simulink model "simu"  (R2025b)
settings: Solver=FixedStepAuto  StartTime=0.0  StopTime=7  FixedStep=0.01  RelTol=1e-3
model workspace (MAT data in the model file):
  T_data = [16.81; 22.34; 22.23; 21.49; 20; 20.21; 18.09; 15.74; 13.4; 10.85; 10.21; 8.94; 8.83; 8.62; 8.62; 8.62; 8.51; 8.72; 8.51; 8.51; 7.77; 7.02; 5.64; 3.83; 2.23; 0.96; 0]
  aero_data.Alpha = [0; 2; 4]
  aero_data.CD = [0.20580088598; 0.20580088598; 0.20580088598]
  aero_data.CL = [0; 0.0625795358549; 0.124860076206]
  aero_data.CP = [0.999; 0.999; 0.999]
  t_data = [0.01; 0.03; 0.11; 0.26; 0.37; 0.47; 0.67; 0.99; 1.31; 1.81; 2.49; 3.13; 3.6; 4.11; 4.95; 5.45; 5.58; 5.88; 6.22; 6.46; 6.6; 6.71; 6.79; 6.91; 6.95; 7; 7.05]
libraries: simulink_extras x2, aerolibatmos2 x1
settings Model: Creator=arjun  LastModifiedBy=piyav

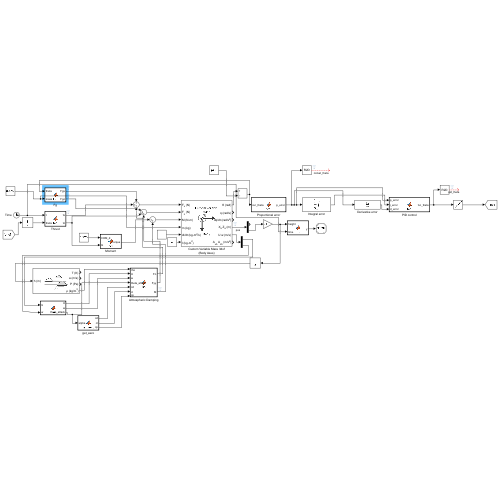
[thumbnail: Simulink's stored preview of the top-level diagram]
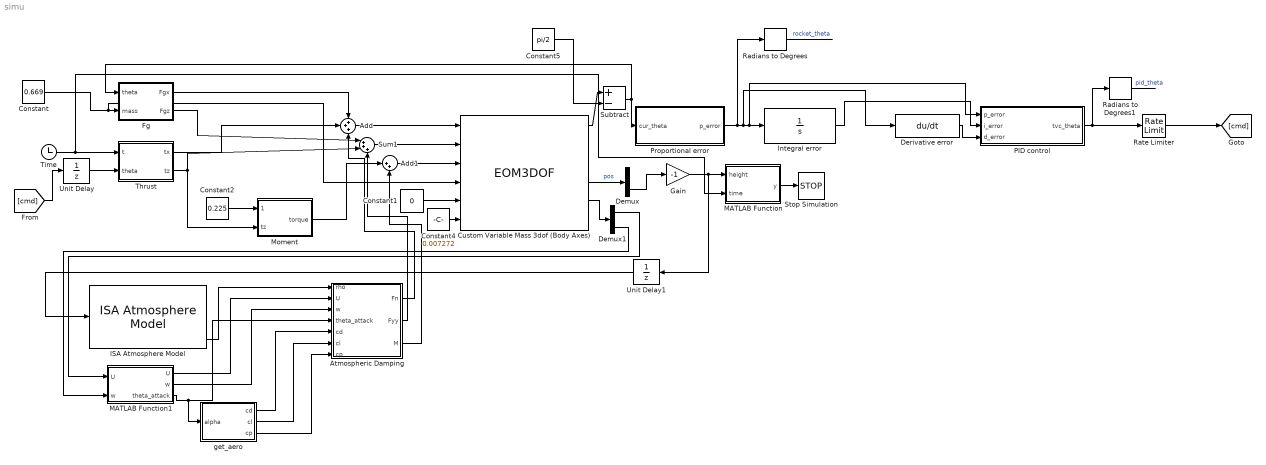
== system simu ==
  Add : Sum  Inputs=+++
  Add1 : Sum  Inputs=|++
  Atmospheric Damping : MATLAB Function  TreatAsAtomicUnit=on
  Constant : Constant  Value=0.669
  Constant1 : Constant  Value=0
  Constant2 : Constant  Value=0.225
  Constant4 : Constant  Value=0.007272  VectorParams1D=off
  Constant5 : Constant  Value=pi/2
  Custom Variable Mass 3dof (Body Axes) : EOM3DOF  mtype=Custom Variable  theta_ini=deg2rad(93)
  Demux : Demux  Outputs=2
  Demux1 : Demux  Outputs=2
  Derivative error : Derivative
  Fg : MATLAB Function  TreatAsAtomicUnit=on
  Gain : Gain  Gain=-1
  ISA Atmosphere Model : aerolibatmos2/ISA Atmosphere Model  useExtended=off  action=Warning  custom=off  viscosityOut=off  g=9.80665  gamma=1.4  R=287.0531  L=0.0065  h_trop=11000  h_strat=20000  rho0=1.225  P0=101325  T0=288.15  h0=0  S=110.4  Tref=273.15  muref=1.716e-5
  Integral error : Integrator  LimitOutput=on  UpperSaturationLimit=0.5  LowerSaturationLimit=-0.5  ContinuousStateAttributes='error'
  MATLAB Function : MATLAB Function  TreatAsAtomicUnit=on
  MATLAB Function1 : MATLAB Function  TreatAsAtomicUnit=on
  Moment : MATLAB Function  TreatAsAtomicUnit=on
  PID control : MATLAB Function  TreatAsAtomicUnit=on
  Proportional error : MATLAB Function  TreatAsAtomicUnit=on
  Radians to Degrees : simulink_extras/Transformations/Radians to Degrees
  Radians to Degrees1 : simulink_extras/Transformations/Radians to Degrees
  Rate Limiter : RateLimiter  RisingSlewLimit=500  FallingSlewLimit=-500  SampleTimeMode=inherited
  Stop Simulation : Stop
  Subtract : Sum  Inputs=+-
  Sum1 : Sum  Inputs=|+++
  Thrust : MATLAB Function  TreatAsAtomicUnit=on
  Time : Clock
  Unit Delay : UnitDelay  InitialCondition=0.0524  SampleTime=-1  HasFrameUpgradeWarning=on
  Unit Delay1 : UnitDelay  SampleTime=-1  HasFrameUpgradeWarning=on
  get_aero : MATLAB Function  TreatAsAtomicUnit=on
  wires:
  Time/1 -> MATLAB Function/2(time), Thrust/1(t)
  Fg/2(Fgz) -> Sum1/1
  Thrust/2(tz) -> Moment/2(tz), Sum1/2
  Sum1/1 -> Custom Variable Mass 3dof (Body Axes)/2
  Add/1 -> Custom Variable Mass 3dof (Body Axes)/1
  Custom Variable Mass 3dof (Body Axes)/4 -> Demux/1  "pos"
  Constant/1 -> Custom Variable Mass 3dof (Body Axes)/4, Fg/2(mass)
  Constant4/1 -> Custom Variable Mass 3dof (Body Axes)/6
  Derivative error/1 -> PID control/3(d_error)
  Integral error/1 -> PID control/2(i_error)
  Proportional error/1(p_error) -> Integral error/1, PID control/1(p_error), Derivative error/1, Radians to Degrees/1
  Constant1/1 -> Custom Variable Mass 3dof (Body Axes)/5
  Radians to Degrees/1 -> ?  "rocket_theta"
  Radians to Degrees1/1 -> ?  "pid_theta"
  Fg/1(Fgx) -> Add/1
  Thrust/1(tx) -> Add/2
  Constant2/1 -> Moment/1(COM_d)
  Demux/2 -> Gain/1
  MATLAB Function/1(y) -> Stop Simulation/1
  Custom Variable Mass 3dof (Body Axes)/5 -> Demux1/1
  Demux1/1 -> MATLAB Function1/1("U ")
  Demux1/2 -> MATLAB Function1/2("w ")
  MATLAB Function1/1(U) -> Atmospheric Damping/2(U)
  MATLAB Function1/2(w) -> Atmospheric Damping/3(w)
  ISA Atmosphere Model/4 -> Atmospheric Damping/1(rho)
  Moment/1(torque) -> Add1/1
  Add1/1 -> Custom Variable Mass 3dof (Body Axes)/3
  MATLAB Function1/3(theta_attack) -> get_aero/1(alpha), Atmospheric Damping/4(theta_attack)
  get_aero/1(cd) -> Atmospheric Damping/5(cd)
  get_aero/2(cl) -> Atmospheric Damping/6(cl)
  get_aero/3(cp) -> Atmospheric Damping/7(cp)
  PID control/1(tvc_theta) -> Rate Limiter/1, Radians to Degrees1/1
  Gain/1 -> MATLAB Function/1(height), Unit Delay1/1
  [cmd] -> Unit Delay/1
  Custom Variable Mass 3dof (Body Axes)/1 -> Subtract/1
  Constant5/1 -> Subtract/2
  Subtract/1 -> Fg/1(theta), Proportional error/1(cur_theta)
  Atmospheric Damping/1(Fn) -> Add/3
  Atmospheric Damping/2(Fyy) -> Sum1/3
  Atmospheric Damping/3(M) -> Add1/2
  Unit Delay1/1 -> ISA Atmosphere Model/1
  Rate Limiter/1 -> [cmd]
  Unit Delay/1 -> Thrust/2(theta)

== matlab function simu/Moment ==
  data: COM_d input; torque output; tz input
function torque = fcn(COM_d, tz)

torque = COM_d * tz;

== matlab function simu/Thrust ==
  data: t input; tx output; tz output; theta input
function [tx, tz] = fcn(t, theta)
    persistent thrust_interp;
    
    if isempty(thrust_interp)
        loadedData = load('interp_thrust_data.mat'); 
        disp(loadedData)
        t_data = loadedData.t_data;
        T_data = loadedData.T_data; 

        thrust_interp = @(t) interp1(t_data, T_data, t, 'pchip', 'extrap');
    end

    burnout_time = 7.246;
    if t < burnout_time
        T = thrust_interp(t);
    else
        T = 0;
    end

    
    tx = T * cos(theta);
    tz = -T * sin(theta);
end

== matlab function simu/MATLAB Function ==
  data: height input; time input; y output
function y = fcn(height, time)

if time > 1 && height < 0
    y = 1;
else
    y = 0;
end

== matlab function simu/Fg ==
  data: theta input; mass input; Fgx output; Fgz output
function [Fgx, Fgz]= fcn(theta, mass)

Fgx = mass * -cos(theta) * 9.8;
Fgz = mass * sin(theta) * -9.8;

== matlab function simu/Proportional error ==
  data: cur_theta input; p_error output
function p_error = fcn(cur_theta)
    p_error = cur_theta;
end

== matlab function simu/PID control ==
  data: p_error input; tvc_theta output; i_error input; d_error input
function tvc_theta = fcn(p_error, i_error, d_error)
    Kp = .4;
    Ki = .15;
    Kd = 0.05;

    tvc_theta = Kp * p_error + Ki * i_error + Kd * d_error;
    tvc_theta = max(min(tvc_theta, deg2rad(7)), -deg2rad(7));
end

== matlab function simu/MATLAB Function1 ==
  data: U output; w output; U input; w input; theta_attack output
function [U, w, theta_attack] = fcn(U, w)

theta_attack = atan(w/U);

== matlab function simu/Atmospheric Damping ==
  data: rho input; Fn output; U input; w input; theta_attack input; cd input; cl input; cp input; Fyy output; M output
function [Fn, Fyy, M] = fcn(rho, U, w, theta_attack, cd, cl, cp)
    V = sqrt(U^2 + w^2);

    Sref = pi * (0.0762/2)^2;

    q = 1/2 * rho * V^2;

    L = q * cl * Sref;
    D = q * cd * Sref;

    Xw = -D;
    Zw = -L;
    
    cg = 0.3302; % from nosecone

    Fn =  cos(theta_attack)*Xw - sin(theta_attack)*Zw
    Fyy =  sin(theta_attack)*Xw + cos(theta_attack)*Zw
    M = Fyy * (cp - cg);
end

== matlab function simu/get_aero ==
  data: alpha input; cd output; cl output; cp output
function [cd, cl, cp] = get_aero(alpha)

    S = load("alpha_interp.mat");  
    Alpha = S.aero_data.Alpha;
    CD_full = S.aero_data.CD;
    CL_full = S.aero_data.CL;
    CP_full = S.aero_data.CP;

    cd = interp1(Alpha, CD_full, alpha, 'linear', 'extrap');
    cl = interp1(Alpha, CL_full, alpha, 'linear', 'extrap');
    cp = interp1(Alpha, CP_full, alpha, 'linear', 'extrap');
    cp = cp * 0.3048;
end
